simulink model "PIcontrolSim"  (R2023a)
settings: Solver=VariableStepAuto  StartTime=0.0  StopTime=10.0  RelTol=1e-3
values from neighbouring files (symbols this model uses):
  b = 50    [PIcontrol.m]    (also in cruiseControl.m; linearModelSim.m)
  Ki = 40    [PIcontrol.m]
  Kp = 800    [PIcontrol.m]
  m = 1000    [PIcontrol.m]    (also in cruiseControl.m; linearModelSim.m)
settings Model: Creator=shrey  LastModifiedBy=shrey

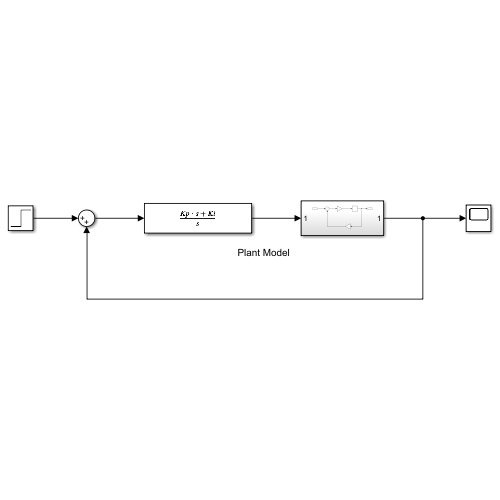
[thumbnail: Simulink's stored preview of the top-level diagram]
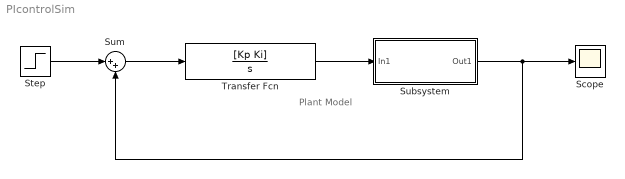
== system PIcontrolSim ==
  note: Plant Model
  Scope : Scope
  Step : Step  Time=0  After=10
  Subsystem : Subsystem
  Sum : Sum  Inputs=|++
  Transfer Fcn : TransferFcn  Numerator=[Kp Ki]  Denominator=[1 0]
  wires:
  Transfer Fcn/1 -> Subsystem/1(In1)
  Step/1 -> Sum/1
  Sum/1 -> Transfer Fcn/1
  Subsystem/1(Out1) -> Sum/2, Scope/1

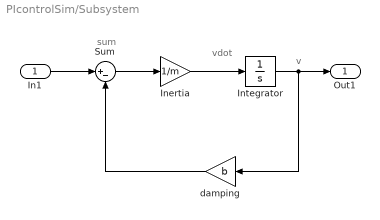
== system PIcontrolSim/Subsystem ==
  note: v
  note: vdot
  note: sum
  In1 : Inport
  Inertia : Gain  Gain=1/m
  Integrator : Integrator
  Sum : Sum  Inputs=|+-
  damping : Gain  Gain=b
  Out1 : Outport
  wires:
  In1/1 -> Sum/1
  Sum/1 -> Inertia/1
  Inertia/1 -> Integrator/1
  Integrator/1 -> Out1/1, damping/1
  damping/1 -> Sum/2
